simulink model "dc_mot_steady_ideal_voltage_without_controller"  (R2019b)
settings: Solver=VariableStepAuto  StartTime=0.0  StopTime=1  RelTol=1e-3
settings Model: Creator=srikesh  LastModifiedBy=srikesh

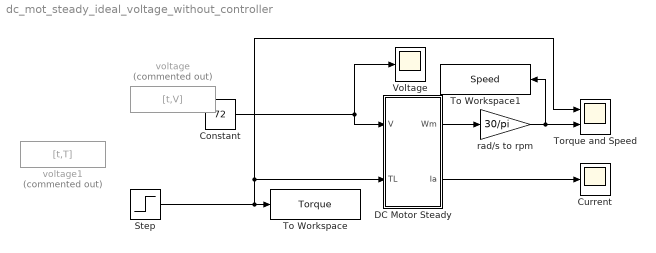
== system dc_mot_steady_ideal_voltage_without_controller ==
  Constant : Constant  Value=72
  Current : Scope
  DC Motor Steady : Subsystem  mask{Ra=.1472, Ke=1.27, Kt=.9852}
      mask prompts: Ra "Ra(Ohm)"; Ke "Ke(V-s)"; Kt "Kt(N-m/A)"
  Step : Step  Time=0  After=20  SampleTime=0
  To Workspace : ToWorkspace  VariableName=Torque  SaveFormat=Timeseries  SampleTime=-1
  To Workspace1 : ToWorkspace  VariableName=Speed  SaveFormat=Timeseries  SampleTime=-1
  Torque and Speed : Scope  NumInputPorts=2
  Voltage : Scope
  "rad/s to rpm " : Gain  Gain=30/pi
  voltage : FromWorkspace  Commented=on  VariableName=[t,V]  SampleTime=0
  voltage1 : FromWorkspace  Commented=on  VariableName=[t,T]  SampleTime=0
  wires:
  DC Motor Steady/1("Wm ") -> "rad/s to rpm "/1
  "rad/s to rpm "/1 -> To Workspace1/1, Torque and Speed/2
  DC Motor Steady/2(Ia) -> Current/1
  Step/1 -> Torque and Speed/1, DC Motor Steady/2("TL "), To Workspace/1
  Constant/1 -> DC Motor Steady/1("V "), Voltage/1

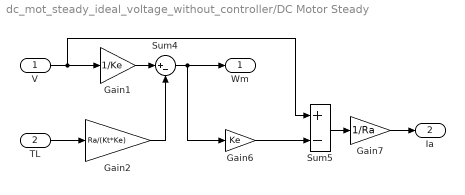
== system dc_mot_steady_ideal_voltage_without_controller/DC Motor Steady ==
  "V " : Inport
  "TL " : Inport  Port=2
  Gain1 : Gain  Gain=1/Ke
  Gain2 : Gain  Gain=Ra/(Kt*Ke)
  Gain6 : Gain  Gain=Ke
  Gain7 : Gain  Gain=1/Ra
  Sum4 : Sum  Inputs=|+-
  Sum5 : Sum  Inputs=+-
  "Wm " : Outport
  Ia : Outport  Port=2
  wires:
  "V "/1 -> Sum5/1, Gain1/1
  Gain1/1 -> Sum4/1
  "TL "/1 -> Gain2/1
  Gain2/1 -> Sum4/2
  Sum4/1 -> Gain6/1, "Wm "/1
  Gain6/1 -> Sum5/2
  Gain7/1 -> Ia/1
  Sum5/1 -> Gain7/1
